simulink model "IEEE30_case"  (R2024b)
settings: Solver=FixedStepAuto  StartTime=0  StopTime=5  FixedStep=1e-7  RelTol=1e-3
values from neighbouring files (symbols this model uses):
  GFL_DFIG_7_C_bus = 0.08    [IEEE30_case_parameters.m]
  GFL_DFIG_7_D_mutual = 2.500000e+3    (= 2500)    [IEEE30_case_parameters.m]
  GFL_DFIG_7_f0 = 60    [IEEE30_case_parameters.m]
  GFL_DFIG_7_gPLLi = 3200    [IEEE30_case_parameters.m]
  GFL_DFIG_7_gPLLp = 650    [IEEE30_case_parameters.m]
  GFL_DFIG_7_H_WT = 0.4    [IEEE30_case_parameters.m]
  GFL_DFIG_7_Hg = 0.8    [IEEE30_case_parameters.m]
  GFL_DFIG_7_Igq_ref = 0    [IEEE30_case_parameters.m]
  GFL_DFIG_7_Ird_ref = 704.45696    [IEEE30_case_parameters.m]
  GFL_DFIG_7_KI_V = -300000    [IEEE30_case_parameters.m]
  GFL_DFIG_7_KP_V = -1000    [IEEE30_case_parameters.m]
  GFL_DFIG_7_Ksh = 1.254300e+4    (= 12543)    [IEEE30_case_parameters.m]
  GFL_DFIG_7_Lg = 0.000483    [IEEE30_case_parameters.m]
  GFL_DFIG_7_Lm_pu = 4    [IEEE30_case_parameters.m]
  GFL_DFIG_7_N = 100    [IEEE30_case_parameters.m]
  GFL_DFIG_7_p = 2    [IEEE30_case_parameters.m]
  GFL_DFIG_7_Pitch = 0    [IEEE30_case_parameters.m]
  GFL_DFIG_7_R = 44    [IEEE30_case_parameters.m]
  GFL_DFIG_7_Rg = 2.000000e-5    (= 2e-05)    [IEEE30_case_parameters.m]
  GFL_DFIG_7_rho = 1.225    [IEEE30_case_parameters.m]
  GFL_DFIG_7_rPLLi = 4500    [IEEE30_case_parameters.m]
  GFL_DFIG_7_rPLLp = 620    [IEEE30_case_parameters.m]
  GFL_DFIG_7_Rs_pu = 0.011    [IEEE30_case_parameters.m]
  GFL_DFIG_7_Sbase = 2.000000e+6    (= 2000000)    [IEEE30_case_parameters.m]
  GFL_DFIG_7_ugq_ref = 0    [IEEE30_case_parameters.m]
  GFL_DFIG_7_usd_ref = 0    [IEEE30_case_parameters.m]
  GFL_DFIG_7_Vbase = 690    [IEEE30_case_parameters.m]
  GFL_DFIG_7_Vdc_ref = 1200    [IEEE30_case_parameters.m]
  GFL_DFIG_7_wind = 12    [IEEE30_case_parameters.m]
  GFL_DFIG_7_wm_ref = 518.184209    [IEEE30_case_parameters.m]
  SG_D_13_D = 0.01056    [IEEE30_case_parameters.m]
  SG_D_13_EnableSaturation = 0    [IEEE30_case_parameters.m]
  SG_D_13_f0 = 60    [IEEE30_case_parameters.m]
  SG_D_13_H = 7.5    [IEEE30_case_parameters.m]
  SG_D_13_K_A = 20    [IEEE30_case_parameters.m]
  SG_D_13_K_E = 1.000000e+1    (= 10)    [IEEE30_case_parameters.m]
  SG_D_13_K_F = 2.363    [IEEE30_case_parameters.m]
  SG_D_13_K_s = 0.5    [IEEE30_case_parameters.m]
  SG_D_13_R_a = 0.001088    [IEEE30_case_parameters.m]
  SG_D_13_S_A = 1    [IEEE30_case_parameters.m]
  SG_D_13_S_B = 0.103    [IEEE30_case_parameters.m]
  SG_D_13_S_N = 10.659857    [IEEE30_case_parameters.m]
  SG_D_13_SpeedPara = 200    [IEEE30_case_parameters.m]
  SG_D_13_T_0 = 0.370163    [IEEE30_case_parameters.m]
  SG_D_13_T_1 = 0.3    [IEEE30_case_parameters.m]
  SG_D_13_T_2 = 0.05    [IEEE30_case_parameters.m]
  SG_D_13_T_3 = 0.02    [IEEE30_case_parameters.m]
  SG_D_13_T_4 = 0.005    [IEEE30_case_parameters.m]
  SG_D_13_T_A = 0.02    [IEEE30_case_parameters.m]
  SG_D_13_T_dd = 8.000000e+0    (= 8)    [IEEE30_case_parameters.m]
  SG_D_13_T_ddd = 0.04    [IEEE30_case_parameters.m]
  SG_D_13_T_E = 0.314    [IEEE30_case_parameters.m]
  SG_D_13_T_F = 0.35    [IEEE30_case_parameters.m]
  SG_D_13_T_qd = 0.8    [IEEE30_case_parameters.m]
  SG_D_13_T_qdd = 0.02    [IEEE30_case_parameters.m]
  SG_D_13_T_speed = 0.1    [IEEE30_case_parameters.m]
  SG_D_13_T_w = 0.5    [IEEE30_case_parameters.m]
  SG_D_13_V_ref = 1.696619    [IEEE30_case_parameters.m]
  SG_D_13_w_ref = 376.991118    [IEEE30_case_parameters.m]
  SG_D_13_x_d = 1.9    [IEEE30_case_parameters.m]
  SG_D_13_x_dd = 0.302    [IEEE30_case_parameters.m]
  SG_D_13_x_ddd = 0.204    [IEEE30_case_parameters.m]
  SG_D_13_x_l = 0.05    [IEEE30_case_parameters.m]
  SG_D_13_x_q = 1.3    [IEEE30_case_parameters.m]
  SG_D_13_x_qd = 0.5    [IEEE30_case_parameters.m]
  SG_D_13_x_qdd = 0.3    [IEEE30_case_parameters.m]
  SG_D_1_D = 0.01056    [IEEE30_case_parameters.m]
  SG_D_1_EnableSaturation = 0    [IEEE30_case_parameters.m]
  SG_D_1_f0 = 60    [IEEE30_case_parameters.m]
  SG_D_1_H = 7.5    [IEEE30_case_parameters.m]
  SG_D_1_K_A = 20    [IEEE30_case_parameters.m]
  SG_D_1_K_E = 1.000000e+1    (= 10)    [IEEE30_case_parameters.m]
  SG_D_1_K_F = 2.363    [IEEE30_case_parameters.m]
  SG_D_1_K_s = 0.5    [IEEE30_case_parameters.m]
  SG_D_1_R_a = 0.001088    [IEEE30_case_parameters.m]
  SG_D_1_S_A = 1    [IEEE30_case_parameters.m]
  SG_D_1_S_B = 0.103    [IEEE30_case_parameters.m]
  SG_D_1_S_N = 10.659857    [IEEE30_case_parameters.m]
  SG_D_1_SpeedPara = 200    [IEEE30_case_parameters.m]
  SG_D_1_T_0 = 0.259812    [IEEE30_case_parameters.m]
  SG_D_1_T_1 = 0.3    [IEEE30_case_parameters.m]
  SG_D_1_T_2 = 0.05    [IEEE30_case_parameters.m]
  SG_D_1_T_3 = 0.02    [IEEE30_case_parameters.m]
  SG_D_1_T_4 = 0.005    [IEEE30_case_parameters.m]
  SG_D_1_T_A = 0.02    [IEEE30_case_parameters.m]
  SG_D_1_T_dd = 8.000000e+0    (= 8)    [IEEE30_case_parameters.m]
  SG_D_1_T_ddd = 0.04    [IEEE30_case_parameters.m]
  SG_D_1_T_E = 0.314    [IEEE30_case_parameters.m]
  SG_D_1_T_F = 0.35    [IEEE30_case_parameters.m]
  SG_D_1_T_qd = 0.8    [IEEE30_case_parameters.m]
  SG_D_1_T_qdd = 0.02    [IEEE30_case_parameters.m]
  SG_D_1_T_speed = 0.1    [IEEE30_case_parameters.m]
  SG_D_1_T_w = 0.5    [IEEE30_case_parameters.m]
  SG_D_1_V_ref = 1.544107    [IEEE30_case_parameters.m]
  SG_D_1_w_ref = 376.991118    [IEEE30_case_parameters.m]
  SG_D_1_x_d = 1.9    [IEEE30_case_parameters.m]
  SG_D_1_x_dd = 0.302    [IEEE30_case_parameters.m]
  SG_D_1_x_ddd = 0.204    [IEEE30_case_parameters.m]
  SG_D_1_x_l = 0.05    [IEEE30_case_parameters.m]
  SG_D_1_x_q = 1.3    [IEEE30_case_parameters.m]
  SG_D_1_x_qd = 0.5    [IEEE30_case_parameters.m]
  SG_D_1_x_qdd = 0.3    [IEEE30_case_parameters.m]
  SG_D_22_D = 0.01056    [IEEE30_case_parameters.m]
  SG_D_22_EnableSaturation = 0    [IEEE30_case_parameters.m]
  SG_D_22_f0 = 60    [IEEE30_case_parameters.m]
  SG_D_22_H = 7.5    [IEEE30_case_parameters.m]
  SG_D_22_K_A = 20    [IEEE30_case_parameters.m]
  SG_D_22_K_E = 1.000000e+1    (= 10)    [IEEE30_case_parameters.m]
  SG_D_22_K_F = 2.363    [IEEE30_case_parameters.m]
  SG_D_22_K_s = 0.5    [IEEE30_case_parameters.m]
  SG_D_22_R_a = 0.001088    [IEEE30_case_parameters.m]
  SG_D_22_S_A = 1    [IEEE30_case_parameters.m]
  SG_D_22_S_B = 0.103    [IEEE30_case_parameters.m]
  SG_D_22_S_N = 10.659857    [IEEE30_case_parameters.m]
  SG_D_22_SpeedPara = 200    [IEEE30_case_parameters.m]
  SG_D_22_T_0 = 0.216121    [IEEE30_case_parameters.m]
  SG_D_22_T_1 = 0.3    [IEEE30_case_parameters.m]
  SG_D_22_T_2 = 0.05    [IEEE30_case_parameters.m]
  SG_D_22_T_3 = 0.02    [IEEE30_case_parameters.m]
  SG_D_22_T_4 = 0.005    [IEEE30_case_parameters.m]
  ... (+126 more)
(part 6 of 27)

== system IEEE30_case/AC_1/d_id_line_5_7_block ==
  note: d_id_line_5_7 in IEEE30_case
      | $376.991118430775\,\mathrm{iq}_{\mathrm{line},5,7}-157.07963267949\,\mathrm{id}_{\mathrm{line},5,7}+3141.59265358979\,\mathrm{vd}_{\mathrm{bus},5}-3141.59265358979\,\mathrm{vd}_{\mathrm{bus},7}$
      | Automatically generated on 2025-11-01 18:41:13 .
  State_id_line_5_7_f4de4 : Inport
  State_iq_line_5_7_abaf2 : Inport  Port=2
  State_vd_bus_5_fcd45 : Inport  Port=3
  State_vd_bus_7_ca274 : Inport  Port=4
  Add_3cebd : Sum
  Add_96d6b : Sum
  Constant_-157.07963267949_79139 : Constant  Value=-157.07963267949
  Constant_3141.59265358979_57f19 : Constant  Value=3141.59265358979
  Constant_3141.59265358979_dc5fb : Constant  Value=3141.59265358979
  Constant_376.991118430775_d7487 : Constant  Value=376.991118430775
  Product_17bef : Product
  Product_21c14 : Product
  Product_bd274 : Product
  Product_f508a : Product
  Subtract_98652 : Sum  Inputs=+-
  Blockout_d_id_line_5_7_7d91d : Outport
  wires:
  Subtract_98652/1 -> Blockout_d_id_line_5_7_7d91d/1
  State_id_line_5_7_f4de4/1 -> Product_17bef/2
  Constant_-157.07963267949_79139/1 -> Product_17bef/1
  Constant_376.991118430775_d7487/1 -> Product_bd274/1
  State_iq_line_5_7_abaf2/1 -> Product_bd274/2
  Product_bd274/1 -> Add_96d6b/2
  Product_17bef/1 -> Add_96d6b/1
  Product_f508a/1 -> Add_3cebd/2
  Constant_3141.59265358979_57f19/1 -> Product_f508a/1
  State_vd_bus_5_fcd45/1 -> Product_f508a/2
  Add_96d6b/1 -> Add_3cebd/1
  Product_21c14/1 -> Subtract_98652/2
  Constant_3141.59265358979_dc5fb/1 -> Product_21c14/1
  State_vd_bus_7_ca274/1 -> Product_21c14/2
  Add_3cebd/1 -> Subtract_98652/1

== system IEEE30_case/AC_1/d_id_line_6_10_block ==
  note: d_id_line_6_10 in IEEE30_case
      | $376.991118430775\,\mathrm{iq}_{\mathrm{line},6,10}+673.198425769241\,\mathrm{vd}_{\mathrm{bus},6}-673.198425769241\,\mathrm{vd}_{\mathrm{bus},10}$
      | Automatically generated on 2025-11-01 18:41:23 .
  State_iq_line_6_10_1e2b8 : Inport
  State_vd_bus_10_6889c : Inport  Port=2
  State_vd_bus_6_f8a31 : Inport  Port=3
  Add_cf162 : Sum
  Constant_376.991118430775_5db38 : Constant  Value=376.991118430775
  Constant_673.198425769241_4baa2 : Constant  Value=673.198425769241
  Constant_673.198425769241_5d573 : Constant  Value=673.198425769241
  Product_2d753 : Product
  Product_3532c : Product
  Product_b0b85 : Product
  Subtract_eeeb7 : Sum  Inputs=+-
  Blockout_d_id_line_6_10_40498 : Outport
  wires:
  Constant_376.991118430775_5db38/1 -> Product_2d753/1
  Constant_673.198425769241_5d573/1 -> Product_b0b85/1
  State_iq_line_6_10_1e2b8/1 -> Product_2d753/2
  Constant_673.198425769241_4baa2/1 -> Product_3532c/1
  Product_3532c/1 -> Subtract_eeeb7/2
  State_vd_bus_10_6889c/1 -> Product_3532c/2
  Product_2d753/1 -> Subtract_eeeb7/1
  State_vd_bus_6_f8a31/1 -> Product_b0b85/2
  Subtract_eeeb7/1 -> Add_cf162/1
  Product_b0b85/1 -> Add_cf162/2
  Add_cf162/1 -> Blockout_d_id_line_6_10_40498/1

== system IEEE30_case/AC_1/d_id_line_6_28_block ==
  note: d_id_line_6_28 in IEEE30_case
      | $376.991118430775\,\mathrm{iq}_{\mathrm{line},6,28}-125.663706143592\,\mathrm{id}_{\mathrm{line},6,28}+6283.18530717959\,\mathrm{vd}_{\mathrm{bus},6}-6283.18530717959\,\mathrm{vd}_{\mathrm{bus},28}$
      | Automatically generated on 2025-11-01 18:42:30 .
  State_id_line_6_28_16dd7 : Inport
  State_iq_line_6_28_4e6de : Inport  Port=2
  State_vd_bus_28_34661 : Inport  Port=3
  State_vd_bus_6_24f43 : Inport  Port=4
  Add_91382 : Sum
  Add_d7cc6 : Sum
  Constant_-125.663706143592_673b1 : Constant  Value=-125.663706143592
  Constant_376.991118430775_83a0d : Constant  Value=376.991118430775
  Constant_6283.18530717959_21113 : Constant  Value=6283.18530717959
  Constant_6283.18530717959_269c0 : Constant  Value=6283.18530717959
  Product_6c6ef : Product
  Product_d631f : Product
  Product_ea0c3 : Product
  Product_ec862 : Product
  Subtract_8b6c5 : Sum  Inputs=+-
  Blockout_d_id_line_6_28_3a173 : Outport
  wires:
  Constant_-125.663706143592_673b1/1 -> Product_d631f/1
  Constant_376.991118430775_83a0d/1 -> Product_ea0c3/1
  Product_ea0c3/1 -> Add_d7cc6/2
  State_id_line_6_28_16dd7/1 -> Product_d631f/2
  Add_91382/1 -> Blockout_d_id_line_6_28_3a173/1
  State_iq_line_6_28_4e6de/1 -> Product_ea0c3/2
  Product_d631f/1 -> Add_d7cc6/1
  Product_6c6ef/1 -> Subtract_8b6c5/2
  Constant_6283.18530717959_269c0/1 -> Product_6c6ef/1
  State_vd_bus_28_34661/1 -> Product_6c6ef/2
  Add_d7cc6/1 -> Subtract_8b6c5/1
  Product_ec862/1 -> Add_91382/2
  Constant_6283.18530717959_21113/1 -> Product_ec862/1
  State_vd_bus_6_24f43/1 -> Product_ec862/2
  Subtract_8b6c5/1 -> Add_91382/1

== system IEEE30_case/AC_1/d_id_line_6_7_block ==
  note: d_id_line_6_7 in IEEE30_case
      | $376.991118430775\,\mathrm{iq}_{\mathrm{line},6,7}-141.371669411541\,\mathrm{id}_{\mathrm{line},6,7}+4712.38898038469\,\mathrm{vd}_{\mathrm{bus},6}-4712.38898038469\,\mathrm{vd}_{\mathrm{bus},7}$
      | Automatically generated on 2025-11-01 18:41:16 .
  State_id_line_6_7_795b3 : Inport
  State_iq_line_6_7_8098b : Inport  Port=2
  State_vd_bus_6_7185e : Inport  Port=3
  State_vd_bus_7_fcdb6 : Inport  Port=4
  Add_20df1 : Sum
  Add_5e0cb : Sum
  Constant_-141.371669411541_b0a47 : Constant  Value=-141.371669411541
  Constant_376.991118430775_4adcf : Constant  Value=376.991118430775
  Constant_4712.38898038469_28790 : Constant  Value=4712.38898038469
  Constant_4712.38898038469_75038 : Constant  Value=4712.38898038469
  Product_b6763 : Product
  Product_dac56 : Product
  Product_e27ef : Product
  Product_fbe98 : Product
  Subtract_3d01d : Sum  Inputs=+-
  Blockout_d_id_line_6_7_5bfdb : Outport
  wires:
  Constant_-141.371669411541_b0a47/1 -> Product_fbe98/1
  State_id_line_6_7_795b3/1 -> Product_fbe98/2
  Constant_376.991118430775_4adcf/1 -> Product_b6763/1
  Product_b6763/1 -> Add_5e0cb/2
  State_iq_line_6_7_8098b/1 -> Product_b6763/2
  Product_fbe98/1 -> Add_5e0cb/1
  Constant_4712.38898038469_28790/1 -> Product_e27ef/1
  State_vd_bus_6_7185e/1 -> Product_e27ef/2
  Add_5e0cb/1 -> Add_20df1/1
  Product_e27ef/1 -> Add_20df1/2
  Product_dac56/1 -> Subtract_3d01d/2
  Constant_4712.38898038469_75038/1 -> Product_dac56/1
  State_vd_bus_7_fcdb6/1 -> Product_dac56/2
  Add_20df1/1 -> Subtract_3d01d/1
  Subtract_3d01d/1 -> Blockout_d_id_line_6_7_5bfdb/1

== system IEEE30_case/AC_1/d_id_line_6_8_block ==
  note: d_id_line_6_8 in IEEE30_case
      | $376.991118430775\,\mathrm{iq}_{\mathrm{line},6,8}-94.2477796076938\,\mathrm{id}_{\mathrm{line},6,8}+9424.77796076938\,\mathrm{vd}_{\mathrm{bus},6}-9424.77796076938\,\mathrm{vd}_{\mathrm{bus},8}$
      | Automatically generated on 2025-11-01 18:41:18 .
  State_id_line_6_8_be2c2 : Inport
  State_iq_line_6_8_15cb0 : Inport  Port=2
  State_vd_bus_6_a2a00 : Inport  Port=3
  State_vd_bus_8_3fe16 : Inport  Port=4
  Add_21824 : Sum
  Add_44597 : Sum
  Constant_-94.2477796076938_c506f : Constant  Value=-94.2477796076938
  Constant_376.991118430775_5cbac : Constant  Value=376.991118430775
  Constant_9424.77796076938_a2f7d : Constant  Value=9424.77796076938
  Constant_9424.77796076938_c3a88 : Constant  Value=9424.77796076938
  Product_448dc : Product
  Product_52dc7 : Product
  Product_5c49d : Product
  Product_d96d0 : Product
  Subtract_76e2a : Sum  Inputs=+-
  Blockout_d_id_line_6_8_230ec : Outport
  wires:
  State_vd_bus_6_a2a00/1 -> Product_448dc/2
  Constant_-94.2477796076938_c506f/1 -> Product_d96d0/1
  Product_448dc/1 -> Add_21824/2
  Constant_9424.77796076938_a2f7d/1 -> Product_448dc/1
  State_id_line_6_8_be2c2/1 -> Product_d96d0/2
  Constant_376.991118430775_5cbac/1 -> Product_52dc7/1
  Product_52dc7/1 -> Add_44597/2
  State_iq_line_6_8_15cb0/1 -> Product_52dc7/2
  Product_5c49d/1 -> Subtract_76e2a/2
  Constant_9424.77796076938_c3a88/1 -> Product_5c49d/1
  Product_d96d0/1 -> Add_44597/1
  Add_44597/1 -> Add_21824/1
  State_vd_bus_8_3fe16/1 -> Product_5c49d/2
  Add_21824/1 -> Subtract_76e2a/1
  Subtract_76e2a/1 -> Blockout_d_id_line_6_8_230ec/1

== system IEEE30_case/AC_1/d_id_line_6_9_block ==
  note: d_id_line_6_9 in IEEE30_case
      | $376.991118430775\,\mathrm{iq}_{\mathrm{line},6,9}+1795.19580205131\,\mathrm{vd}_{\mathrm{bus},6}-1795.19580205131\,\mathrm{vd}_{\mathrm{bus},9}$
      | Automatically generated on 2025-11-01 18:41:21 .
  State_iq_line_6_9_a3af3 : Inport
  State_vd_bus_6_dd441 : Inport  Port=2
  State_vd_bus_9_1e8eb : Inport  Port=3
  Add_a457a : Sum
  Constant_1795.19580205131_21e41 : Constant  Value=1795.19580205131
  Constant_1795.19580205131_4f3db : Constant  Value=1795.19580205131
  Constant_376.991118430775_846aa : Constant  Value=376.991118430775
  Product_8da75 : Product
  Product_af589 : Product
  Product_bd41a : Product
  Subtract_faf1e : Sum  Inputs=+-
  Blockout_d_id_line_6_9_67e91 : Outport
  wires:
  Constant_1795.19580205131_21e41/1 -> Product_8da75/1
  Product_bd41a/1 -> Add_a457a/1
  Constant_376.991118430775_846aa/1 -> Product_bd41a/1
  State_iq_line_6_9_a3af3/1 -> Product_bd41a/2
  Constant_1795.19580205131_4f3db/1 -> Product_af589/1
  Product_af589/1 -> Add_a457a/2
  State_vd_bus_6_dd441/1 -> Product_af589/2
  State_vd_bus_9_1e8eb/1 -> Product_8da75/2
  Add_a457a/1 -> Subtract_faf1e/1
  Product_8da75/1 -> Subtract_faf1e/2
  Subtract_faf1e/1 -> Blockout_d_id_line_6_9_67e91/1

== system IEEE30_case/AC_1/d_id_line_8_28_block ==
  note: d_id_line_8_28 in IEEE30_case
      | $376.991118430775\,\mathrm{iq}_{\mathrm{line},8,28}-113.097335529233\,\mathrm{id}_{\mathrm{line},8,28}+1884.95559215388\,\mathrm{vd}_{\mathrm{bus},8}-1884.95559215388\,\mathrm{vd}_{\mathrm{bus},28}$
      | Automatically generated on 2025-11-01 18:42:27 .
  State_id_line_8_28_e35e6 : Inport
  State_iq_line_8_28_05745 : Inport  Port=2
  State_vd_bus_28_83ac0 : Inport  Port=3
  State_vd_bus_8_26ad6 : Inport  Port=4
  Add_4ec08 : Sum
  Add_5c3f1 : Sum
  Constant_-113.097335529233_90aea : Constant  Value=-113.097335529233
  Constant_1884.95559215388_94dcd : Constant  Value=1884.95559215388
  Constant_1884.95559215388_9cb5d : Constant  Value=1884.95559215388
  Constant_376.991118430775_979c0 : Constant  Value=376.991118430775
  Product_3587f : Product
  Product_8fb7e : Product
  Product_9a9ee : Product
  Product_e88f7 : Product
  Subtract_b3740 : Sum  Inputs=+-
  Blockout_d_id_line_8_28_c2b8a : Outport
  wires:
  Constant_-113.097335529233_90aea/1 -> Product_9a9ee/1
  Constant_1884.95559215388_94dcd/1 -> Product_e88f7/1
  Add_5c3f1/1 -> Blockout_d_id_line_8_28_c2b8a/1
  State_id_line_8_28_e35e6/1 -> Product_9a9ee/2
  Constant_376.991118430775_979c0/1 -> Product_8fb7e/1
  Product_8fb7e/1 -> Add_4ec08/2
  State_iq_line_8_28_05745/1 -> Product_8fb7e/2
  Product_9a9ee/1 -> Add_4ec08/1
  State_vd_bus_28_83ac0/1 -> Product_e88f7/2
  Add_4ec08/1 -> Subtract_b3740/1
  Product_e88f7/1 -> Subtract_b3740/2
  Product_3587f/1 -> Add_5c3f1/2
  Constant_1884.95559215388_9cb5d/1 -> Product_3587f/1
  State_vd_bus_8_26ad6/1 -> Product_3587f/2
  Subtract_b3740/1 -> Add_5c3f1/1

== system IEEE30_case/AC_1/d_id_line_9_10_block ==
  note: d_id_line_9_10 in IEEE30_case
      | $376.991118430775\,\mathrm{iq}_{\mathrm{line},9,10}+3427.19198573432\,\mathrm{vd}_{\mathrm{bus},9}-3427.19198573432\,\mathrm{vd}_{\mathrm{bus},10}$
      | Automatically generated on 2025-11-01 18:41:27 .
  State_iq_line_9_10_60482 : Inport
  State_vd_bus_10_163ea : Inport  Port=2
  State_vd_bus_9_a12d0 : Inport  Port=3
  Add_dcdd8 : Sum
  Constant_3427.19198573432_49acf : Constant  Value=3427.19198573432
  Constant_3427.19198573432_8d0a7 : Constant  Value=3427.19198573432
  Constant_376.991118430775_2c152 : Constant  Value=376.991118430775
  Product_9eddb : Product
  Product_b6cde : Product
  Product_eef34 : Product
  Subtract_03e25 : Sum  Inputs=+-
  Blockout_d_id_line_9_10_c8100 : Outport
  wires:
  State_iq_line_9_10_60482/1 -> Product_9eddb/2
  Constant_376.991118430775_2c152/1 -> Product_9eddb/1
  Constant_3427.19198573432_8d0a7/1 -> Product_eef34/1
  Product_eef34/1 -> Subtract_03e25/2
  State_vd_bus_10_163ea/1 -> Product_eef34/2
  Product_9eddb/1 -> Subtract_03e25/1
  Constant_3427.19198573432_49acf/1 -> Product_b6cde/1
  State_vd_bus_9_a12d0/1 -> Product_b6cde/2
  Subtract_03e25/1 -> Add_dcdd8/1
  Product_b6cde/1 -> Add_dcdd8/2
  Add_dcdd8/1 -> Blockout_d_id_line_9_10_c8100/1

== system IEEE30_case/AC_1/d_id_line_9_11_block ==
  note: d_id_line_9_11 in IEEE30_case
      | $376.991118430775\,\mathrm{iq}_{\mathrm{line},9,11}+1795.19580205131\,\mathrm{vd}_{\mathrm{bus},9}-1795.19580205131\,\mathrm{vd}_{\mathrm{bus},11}$
      | Automatically generated on 2025-11-01 18:41:25 .
  State_iq_line_9_11_d1a32 : Inport
  State_vd_bus_11_30158 : Inport  Port=2
  State_vd_bus_9_653b8 : Inport  Port=3
  Add_d11a9 : Sum
  Constant_1795.19580205131_64bcc : Constant  Value=1795.19580205131
  Constant_1795.19580205131_d59c3 : Constant  Value=1795.19580205131
  Constant_376.991118430775_3b578 : Constant  Value=376.991118430775
  Product_1e074 : Product
  Product_1fdd9 : Product
  Product_4efb2 : Product
  Subtract_8d526 : Sum  Inputs=+-
  Blockout_d_id_line_9_11_6700a : Outport
  wires:
  Constant_376.991118430775_3b578/1 -> Product_4efb2/1
  Constant_1795.19580205131_d59c3/1 -> Product_1fdd9/1
  Product_1fdd9/1 -> Subtract_8d526/2
  State_iq_line_9_11_d1a32/1 -> Product_4efb2/2
  State_vd_bus_11_30158/1 -> Product_1fdd9/2
  Product_4efb2/1 -> Subtract_8d526/1
  Constant_1795.19580205131_64bcc/1 -> Product_1e074/1
  State_vd_bus_9_653b8/1 -> Product_1e074/2
  Subtract_8d526/1 -> Add_d11a9/1
  Product_1e074/1 -> Add_d11a9/2
  Add_d11a9/1 -> Blockout_d_id_line_9_11_6700a/1

== system IEEE30_case/AC_1/d_id_load_10_block ==
  note: d_id_load_10 in IEEE30_case
      | $376.991118430775\,\mathrm{iq}_{\mathrm{load},10}-1093.27424344925\,\mathrm{id}_{\mathrm{load},10}+73.2156181903037\,\mathrm{vd}_{\mathrm{bus},10}$
      | Automatically generated on 2025-11-01 18:40:25 .
  State_id_load_10_b4421 : Inport
  State_iq_load_10_46bbe : Inport  Port=2
  State_vd_bus_10_876fd : Inport  Port=3
  Add_683f6 : Sum
  Add_8289f : Sum
  Constant_-1093.27424344925_8b95d : Constant  Value=-1093.27424344925
  Constant_376.991118430775_85e18 : Constant  Value=376.991118430775
  Constant_73.2156181903037_3ac9c : Constant  Value=73.2156181903037
  Product_21a59 : Product
  Product_23bbe : Product
  Product_24f80 : Product
  Blockout_d_id_load_10_a9a8b : Outport
  wires:
  Constant_-1093.27424344925_8b95d/1 -> Product_24f80/1
  Constant_376.991118430775_85e18/1 -> Product_21a59/1
  Product_21a59/1 -> Add_8289f/2
  Product_24f80/1 -> Add_8289f/1
  State_id_load_10_b4421/1 -> Product_24f80/2
  State_iq_load_10_46bbe/1 -> Product_21a59/2
  Product_23bbe/1 -> Add_683f6/2
  Constant_73.2156181903037_3ac9c/1 -> Product_23bbe/1
  State_vd_bus_10_876fd/1 -> Product_23bbe/2
  Add_8289f/1 -> Add_683f6/1
  Add_683f6/1 -> Blockout_d_id_load_10_a9a8b/1

== system IEEE30_case/AC_1/d_id_load_12_block ==
  note: d_id_load_12 in IEEE30_case
      | $376.991118430775\,\mathrm{iq}_{\mathrm{load},12}-562.973403523291\,\mathrm{id}_{\mathrm{load},12}+94.0406333232708\,\mathrm{vd}_{\mathrm{bus},12}$
      | Automatically generated on 2025-11-01 18:40:27 .
  State_id_load_12_7246e : Inport
  State_iq_load_12_5d0f3 : Inport  Port=2
  State_vd_bus_12_e073f : Inport  Port=3
  Add_15efc : Sum
  Add_f0d24 : Sum
  Constant_-562.973403523291_16ce0 : Constant  Value=-562.973403523291
  Constant_376.991118430775_26874 : Constant  Value=376.991118430775
  Constant_94.0406333232708_30ced : Constant  Value=94.0406333232708
  Product_2d4c6 : Product
  Product_385f8 : Product
  Product_9dcd7 : Product
  Blockout_d_id_load_12_82ad0 : Outport
  wires:
  Constant_-562.973403523291_16ce0/1 -> Product_385f8/1
  Product_385f8/1 -> Add_15efc/1
  State_id_load_12_7246e/1 -> Product_385f8/2
  Constant_376.991118430775_26874/1 -> Product_9dcd7/1
  Product_9dcd7/1 -> Add_15efc/2
  State_iq_load_12_5d0f3/1 -> Product_9dcd7/2
  Product_2d4c6/1 -> Add_f0d24/2
  Constant_94.0406333232708_30ced/1 -> Product_2d4c6/1
  State_vd_bus_12_e073f/1 -> Product_2d4c6/2
  Add_15efc/1 -> Add_f0d24/1
  Add_f0d24/1 -> Blockout_d_id_load_12_82ad0/1

== system IEEE30_case/AC_1/d_id_load_14_block ==
  note: d_id_load_14 in IEEE30_case
      | $376.991118430775\,\mathrm{iq}_{\mathrm{load},14}-1460.84058391925\,\mathrm{id}_{\mathrm{load},14}+101.272894526084\,\mathrm{vd}_{\mathrm{bus},14}$
      | Automatically generated on 2025-11-01 18:40:30 .
  State_id_load_14_cc3a3 : Inport
  State_iq_load_14_d649f : Inport  Port=2
  State_vd_bus_14_f08fd : Inport  Port=3
  Add_0838c : Sum
  Add_4ad40 : Sum
  Constant_-1460.84058391925_2a859 : Constant  Value=-1460.84058391925
  Constant_101.272894526084_890bb : Constant  Value=101.272894526084
  Constant_376.991118430775_aab37 : Constant  Value=376.991118430775
  Product_31438 : Product
  Product_944f5 : Product
  Product_a5863 : Product
  Blockout_d_id_load_14_6d751 : Outport
  wires:
  Constant_-1460.84058391925_2a859/1 -> Product_31438/1
  Product_31438/1 -> Add_4ad40/1
  State_id_load_14_cc3a3/1 -> Product_31438/2
  Constant_376.991118430775_aab37/1 -> Product_944f5/1
  Product_944f5/1 -> Add_4ad40/2
  Product_a5863/1 -> Add_0838c/2
  Constant_101.272894526084_890bb/1 -> Product_a5863/1
  State_iq_load_14_d649f/1 -> Product_944f5/2
  Add_0838c/1 -> Blockout_d_id_load_14_6d751/1
  State_vd_bus_14_f08fd/1 -> Product_a5863/2
  Add_4ad40/1 -> Add_0838c/1

== system IEEE30_case/AC_1/d_id_load_15_block ==
  note: d_id_load_15 in IEEE30_case
      | $376.991118430775\,\mathrm{iq}_{\mathrm{load},15}-1236.53086845294\,\mathrm{id}_{\mathrm{load},15}+115.335827789783\,\mathrm{vd}_{\mathrm{bus},15}$
      | Automatically generated on 2025-11-01 18:40:32 .
  State_id_load_15_eb719 : Inport
  State_iq_load_15_a3946 : Inport  Port=2
  State_vd_bus_15_8a842 : Inport  Port=3
  Add_5f190 : Sum
  Add_ffceb : Sum
  Constant_-1236.53086845294_1de0b : Constant  Value=-1236.53086845294
  Constant_115.335827789783_e0e0e : Constant  Value=115.335827789783
  Constant_376.991118430775_a00d5 : Constant  Value=376.991118430775
  Product_d7855 : Product
  Product_d9c37 : Product
  Product_f5b16 : Product
  Blockout_d_id_load_15_10a9e : Outport
  wires:
  State_vd_bus_15_8a842/1 -> Product_f5b16/2
  Add_ffceb/1 -> Add_5f190/1
  Constant_-1236.53086845294_1de0b/1 -> Product_d7855/1
  Product_f5b16/1 -> Add_5f190/2
  Constant_115.335827789783_e0e0e/1 -> Product_f5b16/1
  Product_d7855/1 -> Add_ffceb/1
  State_id_load_15_eb719/1 -> Product_d7855/2
  Constant_376.991118430775_a00d5/1 -> Product_d9c37/1
  Product_d9c37/1 -> Add_ffceb/2
  State_iq_load_15_a3946/1 -> Product_d9c37/2
  Add_5f190/1 -> Blockout_d_id_load_15_10a9e/1

== system IEEE30_case/AC_1/d_id_load_16_block ==
  note: d_id_load_16 in IEEE30_case
      | $376.991118430775\,\mathrm{iq}_{\mathrm{load},16}-733.038285837618\,\mathrm{id}_{\mathrm{load},16}+33.9601202098734\,\mathrm{vd}_{\mathrm{bus},16}$
      | Automatically generated on 2025-11-01 18:40:34 .
  State_id_load_16_b19cd : Inport
  State_iq_load_16_b414b : Inport  Port=2
  State_vd_bus_16_dbff6 : Inport  Port=3
  Add_04344 : Sum
  Add_c11be : Sum
  Constant_-733.038285837618_5814f : Constant  Value=-733.038285837618
  Constant_33.9601202098734_4dcff : Constant  Value=33.9601202098734
  Constant_376.991118430775_a0c4a : Constant  Value=376.991118430775
  Product_052c1 : Product
  Product_a73ff : Product
  Product_e285b : Product
  Blockout_d_id_load_16_4c50d : Outport
  wires:
  Constant_-733.038285837618_5814f/1 -> Product_a73ff/1
  Constant_376.991118430775_a0c4a/1 -> Product_052c1/1
  Product_052c1/1 -> Add_c11be/2
  Product_a73ff/1 -> Add_c11be/1
  State_id_load_16_b19cd/1 -> Product_a73ff/2
  State_iq_load_16_b414b/1 -> Product_052c1/2
  Product_e285b/1 -> Add_04344/2
  Constant_33.9601202098734_4dcff/1 -> Product_e285b/1
  Add_04344/1 -> Blockout_d_id_load_16_4c50d/1
  State_vd_bus_16_dbff6/1 -> Product_e285b/2
  Add_c11be/1 -> Add_04344/1

== system IEEE30_case/AC_1/d_id_load_17_block ==
  note: d_id_load_17 in IEEE30_case
      | $376.991118430775\,\mathrm{iq}_{\mathrm{load},17}-584.986218254651\,\mathrm{id}_{\mathrm{load},17}+78.0853999068988\,\mathrm{vd}_{\mathrm{bus},17}$
      | Automatically generated on 2025-11-01 18:40:36 .
  State_id_load_17_a4ece : Inport
  State_iq_load_17_ca59a : Inport  Port=2
  State_vd_bus_17_34bc4 : Inport  Port=3
  Add_b66f2 : Sum
  Add_f0f0b : Sum
  Constant_-584.986218254651_7f0eb : Constant  Value=-584.986218254651
  Constant_376.991118430775_c7146 : Constant  Value=376.991118430775
  Constant_78.0853999068988_505df : Constant  Value=78.0853999068988
  Product_113aa : Product
  Product_75b41 : Product
  Product_d00df : Product
  Blockout_d_id_load_17_000e5 : Outport
  wires:
  Constant_-584.986218254651_7f0eb/1 -> Product_75b41/1
  Product_75b41/1 -> Add_b66f2/1
  State_id_load_17_a4ece/1 -> Product_75b41/2
  Constant_376.991118430775_c7146/1 -> Product_d00df/1
  Product_d00df/1 -> Add_b66f2/2
  State_iq_load_17_ca59a/1 -> Product_d00df/2
  Product_113aa/1 -> Add_f0f0b/2
  Constant_78.0853999068988_505df/1 -> Product_113aa/1
  State_vd_bus_17_34bc4/1 -> Product_113aa/2
  Add_b66f2/1 -> Add_f0f0b/1
  Add_f0f0b/1 -> Blockout_d_id_load_17_000e5/1

== system IEEE30_case/AC_1/d_id_load_18_block ==
  note: d_id_load_18 in IEEE30_case
      | $376.991118430775\,\mathrm{iq}_{\mathrm{load},18}-1340.41286553164\,\mathrm{id}_{\mathrm{load},18}+49.3520450041255\,\mathrm{vd}_{\mathrm{bus},18}$
      | Automatically generated on 2025-11-01 18:40:38 .
  State_id_load_18_c255f : Inport
  State_iq_load_18_e520e : Inport  Port=2
  State_vd_bus_18_bf8f3 : Inport  Port=3
  Add_045e5 : Sum
  Add_5e28f : Sum
  Constant_-1340.41286553164_81c67 : Constant  Value=-1340.41286553164
  Constant_376.991118430775_9c70f : Constant  Value=376.991118430775
  Constant_49.3520450041255_59f5b : Constant  Value=49.3520450041255
  Product_50b44 : Product
  Product_a97c5 : Product
  Product_c1ec3 : Product
  Blockout_d_id_load_18_3083b : Outport
  wires:
  Constant_-1340.41286553164_81c67/1 -> Product_a97c5/1
  Product_a97c5/1 -> Add_5e28f/1
  State_id_load_18_c255f/1 -> Product_a97c5/2
  Constant_376.991118430775_9c70f/1 -> Product_c1ec3/1
  Product_c1ec3/1 -> Add_5e28f/2
  Product_50b44/1 -> Add_045e5/2
  Constant_49.3520450041255_59f5b/1 -> Product_50b44/1
  State_iq_load_18_e520e/1 -> Product_c1ec3/2
  State_vd_bus_18_bf8f3/1 -> Product_50b44/2
  Add_5e28f/1 -> Add_045e5/1
  Add_045e5/1 -> Blockout_d_id_load_18_3083b/1

== system IEEE30_case/AC_1/d_id_load_19_block ==
  note: d_id_load_19 in IEEE30_case
      | $376.991118430775\,\mathrm{iq}_{\mathrm{load},19}-1053.35753679187\,\mathrm{id}_{\mathrm{load},19}+121.151749063551\,\mathrm{vd}_{\mathrm{bus},19}$
      | Automatically generated on 2025-11-01 18:40:40 .
  State_id_load_19_86caa : Inport
  State_iq_load_19_76cc3 : Inport  Port=2
  State_vd_bus_19_07a12 : Inport  Port=3
  Add_39f41 : Sum
  Add_8d624 : Sum
  Constant_-1053.35753679187_bafe0 : Constant  Value=-1053.35753679187
  Constant_121.151749063551_084ae : Constant  Value=121.151749063551
  Constant_376.991118430775_456e5 : Constant  Value=376.991118430775
  Product_003ce : Product
  Product_1d94f : Product
  Product_8f6a5 : Product
  Blockout_d_id_load_19_c7816 : Outport
  wires:
  State_vd_bus_19_07a12/1 -> Product_8f6a5/2
  Constant_-1053.35753679187_bafe0/1 -> Product_1d94f/1
  Product_8f6a5/1 -> Add_8d624/2
  Constant_121.151749063551_084ae/1 -> Product_8f6a5/1
  Product_1d94f/1 -> Add_39f41/1
  State_id_load_19_86caa/1 -> Product_1d94f/2
  Constant_376.991118430775_456e5/1 -> Product_003ce/1
  Product_003ce/1 -> Add_39f41/2
  State_iq_load_19_76cc3/1 -> Product_003ce/2
  Add_39f41/1 -> Add_8d624/1
  Add_8d624/1 -> Blockout_d_id_load_19_c7816/1

== system IEEE30_case/AC_1/d_id_load_20_block ==
  note: d_id_load_20 in IEEE30_case
      | $376.991118430775\,\mathrm{iq}_{\mathrm{load},20}-1184.82922935387\,\mathrm{id}_{\mathrm{load},20}+30.5607236833912\,\mathrm{vd}_{\mathrm{bus},20}$
      | Automatically generated on 2025-11-01 18:40:42 .
  State_id_load_20_93d05 : Inport
  State_iq_load_20_02020 : Inport  Port=2
  State_vd_bus_20_a40d3 : Inport  Port=3
  Add_3d016 : Sum
  Add_73b62 : Sum
  Constant_-1184.82922935387_94f65 : Constant  Value=-1184.82922935387
  Constant_30.5607236833912_571fa : Constant  Value=30.5607236833912
  Constant_376.991118430775_c13cd : Constant  Value=376.991118430775
  Product_3ef52 : Product
  Product_51416 : Product
  Product_7406c : Product
  Blockout_d_id_load_20_0f852 : Outport
  wires:
  Constant_-1184.82922935387_94f65/1 -> Product_51416/1
  Constant_376.991118430775_c13cd/1 -> Product_3ef52/1
  Product_3ef52/1 -> Add_73b62/2
  Product_51416/1 -> Add_73b62/1
  State_id_load_20_93d05/1 -> Product_51416/2
  State_iq_load_20_02020/1 -> Product_3ef52/2
  Product_7406c/1 -> Add_3d016/2
  Constant_30.5607236833912_571fa/1 -> Product_7406c/1
  Add_3d016/1 -> Blockout_d_id_load_20_0f852/1
  State_vd_bus_20_a40d3/1 -> Product_7406c/2
  Add_73b62/1 -> Add_3d016/1

== system IEEE30_case/AC_1/d_id_load_21_block ==
  note: d_id_load_21 in IEEE30_case
      | $376.991118430775\,\mathrm{iq}_{\mathrm{load},21}-589.048622548086\,\mathrm{id}_{\mathrm{load},21}+147.248668081812\,\mathrm{vd}_{\mathrm{bus},21}$
      | Automatically generated on 2025-11-01 18:40:44 .
  State_id_load_21_69a18 : Inport
  State_iq_load_21_49e98 : Inport  Port=2
  State_vd_bus_21_5dea6 : Inport  Port=3
  Add_80ae7 : Sum
  Add_a054e : Sum
  Constant_-589.048622548086_4f999 : Constant  Value=-589.048622548086
  Constant_147.248668081812_4d1f4 : Constant  Value=147.248668081812
  Constant_376.991118430775_edf1b : Constant  Value=376.991118430775
  Product_106cf : Product
  Product_1caf2 : Product
  Product_768ed : Product
  Blockout_d_id_load_21_f09db : Outport
  wires:
  Constant_-589.048622548086_4f999/1 -> Product_768ed/1
  Product_768ed/1 -> Add_80ae7/1
  State_id_load_21_69a18/1 -> Product_768ed/2
  Constant_376.991118430775_edf1b/1 -> Product_106cf/1
  Product_106cf/1 -> Add_80ae7/2
  State_iq_load_21_49e98/1 -> Product_106cf/2
  Product_1caf2/1 -> Add_a054e/2
  Constant_147.248668081812_4d1f4/1 -> Product_1caf2/1
  State_vd_bus_21_5dea6/1 -> Product_1caf2/2
  Add_80ae7/1 -> Add_a054e/1
  Add_a054e/1 -> Blockout_d_id_load_21_f09db/1

== system IEEE30_case/AC_1/d_id_load_23_block ==
  note: d_id_load_23 in IEEE30_case
      | $376.991118430775\,\mathrm{iq}_{\mathrm{load},23}-753.98223686155\,\mathrm{id}_{\mathrm{load},23}+30.159289474462\,\mathrm{vd}_{\mathrm{bus},23}$
      | Automatically generated on 2025-11-01 18:40:46 .
  State_id_load_23_139dd : Inport
  State_iq_load_23_9ed9d : Inport  Port=2
  State_vd_bus_23_3d25c : Inport  Port=3
  Add_cb4a1 : Sum
  Add_fda1a : Sum
  Constant_-753.98223686155_779b8 : Constant  Value=-753.98223686155
  Constant_30.159289474462_e23cc : Constant  Value=30.159289474462
  Constant_376.991118430775_7c271 : Constant  Value=376.991118430775
  Product_85ff3 : Product
  Product_e9dc7 : Product
  Product_f749f : Product
  Blockout_d_id_load_23_0d04d : Outport
  wires:
  Constant_-753.98223686155_779b8/1 -> Product_85ff3/1
  Product_85ff3/1 -> Add_cb4a1/1
  State_id_load_23_139dd/1 -> Product_85ff3/2
  Constant_376.991118430775_7c271/1 -> Product_e9dc7/1
  Product_e9dc7/1 -> Add_cb4a1/2
  Product_f749f/1 -> Add_fda1a/2
  Constant_30.159289474462_e23cc/1 -> Product_f749f/1
  State_iq_load_23_9ed9d/1 -> Product_e9dc7/2
  State_vd_bus_23_3d25c/1 -> Product_f749f/2
  Add_fda1a/1 -> Blockout_d_id_load_23_0d04d/1
  Add_cb4a1/1 -> Add_fda1a/1

== system IEEE30_case/AC_1/d_id_load_24_block ==
  note: d_id_load_24 in IEEE30_case
      | $376.991118430775\,\mathrm{iq}_{\mathrm{load},24}-489.525780648917\,\mathrm{id}_{\mathrm{load},24}+69.4256561190419\,\mathrm{vd}_{\mathrm{bus},24}$
      | Automatically generated on 2025-11-01 18:40:48 .
  State_id_load_24_1ae10 : Inport
  State_iq_load_24_33ce7 : Inport  Port=2
  State_vd_bus_24_e8709 : Inport  Port=3
  Add_2b358 : Sum
  Add_f3861 : Sum
  Constant_-489.525780648917_3d885 : Constant  Value=-489.525780648917
  Constant_376.991118430775_5f561 : Constant  Value=376.991118430775
  Constant_69.4256561190419_6c15a : Constant  Value=69.4256561190419
  Product_11a3b : Product
  Product_24c41 : Product
  Product_5935c : Product
  Blockout_d_id_load_24_7bbe2 : Outport
  wires:
  State_vd_bus_24_e8709/1 -> Product_11a3b/2
  Constant_-489.525780648917_3d885/1 -> Product_24c41/1
  Product_11a3b/1 -> Add_2b358/2
  Constant_69.4256561190419_6c15a/1 -> Product_11a3b/1
  Product_24c41/1 -> Add_f3861/1
  State_id_load_24_1ae10/1 -> Product_24c41/2
  Constant_376.991118430775_5f561/1 -> Product_5935c/1
  Product_5935c/1 -> Add_f3861/2
  State_iq_load_24_33ce7/1 -> Product_5935c/2
  Add_f3861/1 -> Add_2b358/1
  Add_2b358/1 -> Blockout_d_id_load_24_7bbe2/1

== system IEEE30_case/AC_1/d_id_load_26_block ==
  note: d_id_load_26 in IEEE30_case
      | $376.991118430775\,\mathrm{iq}_{\mathrm{load},26}-573.682136742484\,\mathrm{id}_{\mathrm{load},26}+30.4177344988829\,\mathrm{vd}_{\mathrm{bus},26}$
      | Automatically generated on 2025-11-01 18:40:50 .
  State_id_load_26_7d329 : Inport
  State_iq_load_26_8de5f : Inport  Port=2
  State_vd_bus_26_1ef7d : Inport  Port=3
  Add_a8ac2 : Sum
  Add_ab0a7 : Sum
  Constant_-573.682136742484_70732 : Constant  Value=-573.682136742484
  Constant_30.4177344988829_4842c : Constant  Value=30.4177344988829
  Constant_376.991118430775_fb0b4 : Constant  Value=376.991118430775
  Product_3e15b : Product
  Product_4fa69 : Product
  Product_c716b : Product
  Blockout_d_id_load_26_29eef : Outport
  wires:
  Constant_-573.682136742484_70732/1 -> Product_4fa69/1
  Constant_376.991118430775_fb0b4/1 -> Product_c716b/1
  Product_c716b/1 -> Add_a8ac2/2
  Product_4fa69/1 -> Add_a8ac2/1
  State_id_load_26_7d329/1 -> Product_4fa69/2
  State_iq_load_26_8de5f/1 -> Product_c716b/2
  Product_3e15b/1 -> Add_ab0a7/2
  Constant_30.4177344988829_4842c/1 -> Product_3e15b/1
  State_vd_bus_26_1ef7d/1 -> Product_3e15b/2
  Add_a8ac2/1 -> Add_ab0a7/1
  Add_ab0a7/1 -> Blockout_d_id_load_26_29eef/1

== system IEEE30_case/AC_1/d_id_load_29_block ==
  note: d_id_load_29 in IEEE30_case
      | $376.991118430775\,\mathrm{iq}_{\mathrm{load},29}-1005.30964914873\,\mathrm{id}_{\mathrm{load},29}+28.6786928048477\,\mathrm{vd}_{\mathrm{bus},29}$
      | Automatically generated on 2025-11-01 18:40:52 .
  State_id_load_29_75998 : Inport
  State_iq_load_29_726f9 : Inport  Port=2
  State_vd_bus_29_01a46 : Inport  Port=3
  Add_096fd : Sum
  Add_c4333 : Sum
  Constant_-1005.30964914873_4c6ee : Constant  Value=-1005.30964914873
  Constant_28.6786928048477_c193b : Constant  Value=28.6786928048477
  Constant_376.991118430775_3c60a : Constant  Value=376.991118430775
  Product_6b013 : Product
  Product_791a8 : Product
  Product_c42d3 : Product
  Blockout_d_id_load_29_ee930 : Outport
  wires:
  Add_096fd/1 -> Add_c4333/1
  Constant_-1005.30964914873_4c6ee/1 -> Product_c42d3/1
  Product_c42d3/1 -> Add_096fd/1
  State_id_load_29_75998/1 -> Product_c42d3/2
  Constant_376.991118430775_3c60a/1 -> Product_791a8/1
  Product_791a8/1 -> Add_096fd/2
  State_iq_load_29_726f9/1 -> Product_791a8/2
  Product_6b013/1 -> Add_c4333/2
  Constant_28.6786928048477_c193b/1 -> Product_6b013/1
  State_vd_bus_29_01a46/1 -> Product_6b013/2
  Add_c4333/1 -> Blockout_d_id_load_29_ee930/1

== system IEEE30_case/AC_1/d_id_load_2_block ==
  note: d_id_load_2 in IEEE30_case
      | $376.991118430775\,\mathrm{iq}_{\mathrm{load},2}-644.150178736049\,\mathrm{id}_{\mathrm{load},2}+187.658460826431\,\mathrm{vd}_{\mathrm{bus},2}$
      | Automatically generated on 2025-11-01 18:40:14 .
  State_id_load_2_b9eb3 : Inport
  State_iq_load_2_16be9 : Inport  Port=2
  State_vd_bus_2_46ad8 : Inport  Port=3
  Add_0a498 : Sum
  Add_c8c31 : Sum
  Constant_-644.150178736049_6a6d4 : Constant  Value=-644.150178736049
  Constant_187.658460826431_55d7c : Constant  Value=187.658460826431
  Constant_376.991118430775_2d4f7 : Constant  Value=376.991118430775
  Product_03ad6 : Product
  Product_a3185 : Product
  Product_f3371 : Product
  Blockout_d_id_load_2_a0af3 : Outport
  wires:
  State_vd_bus_2_46ad8/1 -> Product_a3185/2
  Constant_-644.150178736049_6a6d4/1 -> Product_03ad6/1
  Product_03ad6/1 -> Add_0a498/1
  Product_a3185/1 -> Add_c8c31/2
  Constant_187.658460826431_55d7c/1 -> Product_a3185/1
  State_id_load_2_b9eb3/1 -> Product_03ad6/2
  Constant_376.991118430775_2d4f7/1 -> Product_f3371/1
  Product_f3371/1 -> Add_0a498/2
  State_iq_load_2_16be9/1 -> Product_f3371/2
  Add_0a498/1 -> Add_c8c31/1
  Add_c8c31/1 -> Blockout_d_id_load_2_a0af3/1

== system IEEE30_case/AC_1/d_id_load_30_block ==
  note: d_id_load_30 in IEEE30_case
      | $376.991118430775\,\mathrm{iq}_{\mathrm{load},30}-2103.21360808748\,\mathrm{id}_{\mathrm{load},30}+245.627822821845\,\mathrm{vd}_{\mathrm{bus},30}$
      | Automatically generated on 2025-11-01 18:40:54 .
  State_id_load_30_f5eec : Inport
  State_iq_load_30_241a5 : Inport  Port=2
  State_vd_bus_30_c111a : Inport  Port=3
  Add_b54c5 : Sum
  Add_f898c : Sum
  Constant_-2103.21360808748_a3447 : Constant  Value=-2103.21360808748
  Constant_245.627822821845_0e239 : Constant  Value=245.627822821845
  Constant_376.991118430775_fc958 : Constant  Value=376.991118430775
  Product_5ed96 : Product
  Product_700f9 : Product
  Product_a45fa : Product
  Blockout_d_id_load_30_6a7a7 : Outport
  wires:
  Constant_-2103.21360808748_a3447/1 -> Product_a45fa/1
  Constant_376.991118430775_fc958/1 -> Product_5ed96/1
  Product_5ed96/1 -> Add_b54c5/2
  Product_a45fa/1 -> Add_b54c5/1
  State_id_load_30_f5eec/1 -> Product_a45fa/2
  State_iq_load_30_241a5/1 -> Product_5ed96/2
  Product_700f9/1 -> Add_f898c/2
  Constant_245.627822821845_0e239/1 -> Product_700f9/1
  Add_f898c/1 -> Blockout_d_id_load_30_6a7a7/1
  State_vd_bus_30_c111a/1 -> Product_700f9/2
  Add_b54c5/1 -> Add_f898c/1

== system IEEE30_case/AC_1/d_id_load_3_block ==
  note: d_id_load_3 in IEEE30_case
      | $376.991118430775\,\mathrm{iq}_{\mathrm{load},3}-753.98223686155\,\mathrm{id}_{\mathrm{load},3}+23.4020092990225\,\mathrm{vd}_{\mathrm{bus},3}$
      | Automatically generated on 2025-11-01 18:40:17 .
  State_id_load_3_6ca3f : Inport
  State_iq_load_3_e3dcb : Inport  Port=2
  State_vd_bus_3_703c2 : Inport  Port=3
  Add_a2206 : Sum
  Add_e9327 : Sum
  Constant_-753.98223686155_27bf7 : Constant  Value=-753.98223686155
  Constant_23.4020092990225_cfb13 : Constant  Value=23.4020092990225
  Constant_376.991118430775_2770c : Constant  Value=376.991118430775
  Product_30cb6 : Product
  Product_5007e : Product
  Product_59e16 : Product
  Blockout_d_id_load_3_d01d9 : Outport
  wires:
  Constant_-753.98223686155_27bf7/1 -> Product_5007e/1
  Constant_376.991118430775_2770c/1 -> Product_30cb6/1
  Product_30cb6/1 -> Add_a2206/2
  Product_5007e/1 -> Add_a2206/1
  State_id_load_3_6ca3f/1 -> Product_5007e/2
  State_iq_load_3_e3dcb/1 -> Product_30cb6/2
  Product_59e16/1 -> Add_e9327/2
  Constant_23.4020092990225_cfb13/1 -> Product_59e16/1
  State_vd_bus_3_703c2/1 -> Product_59e16/2
  Add_a2206/1 -> Add_e9327/1
  Add_e9327/1 -> Blockout_d_id_load_3_d01d9/1

== system IEEE30_case/AC_1/d_id_load_4_block ==
  note: d_id_load_4 in IEEE30_case
      | $376.991118430775\,\mathrm{iq}_{\mathrm{load},4}-1790.70781254618\,\mathrm{id}_{\mathrm{load},4}+147.957809890804\,\mathrm{vd}_{\mathrm{bus},4}$
      | Automatically generated on 2025-11-01 18:40:19 .
  State_id_load_4_a067e : Inport
  State_iq_load_4_59598 : Inport  Port=2
  State_vd_bus_4_a96c2 : Inport  Port=3
  Add_28b14 : Sum
  Add_2e701 : Sum
  Constant_-1790.70781254618_4a751 : Constant  Value=-1790.70781254618
  Constant_147.957809890804_b436d : Constant  Value=147.957809890804
  Constant_376.991118430775_a92b6 : Constant  Value=376.991118430775
  Product_6b4e9 : Product
  Product_ee5ea : Product
  Product_f31c8 : Product
  Blockout_d_id_load_4_41d2b : Outport
  wires:
  Add_28b14/1 -> Add_2e701/1
  Constant_-1790.70781254618_4a751/1 -> Product_f31c8/1
  Product_f31c8/1 -> Add_28b14/1
  State_id_load_4_a067e/1 -> Product_f31c8/2
  Constant_376.991118430775_a92b6/1 -> Product_ee5ea/1
  Product_ee5ea/1 -> Add_28b14/2
  State_iq_load_4_59598/1 -> Product_ee5ea/2
  Product_6b4e9/1 -> Add_2e701/2
  Constant_147.957809890804_b436d/1 -> Product_6b4e9/1
  State_vd_bus_4_a96c2/1 -> Product_6b4e9/2
  Add_2e701/1 -> Blockout_d_id_load_4_41d2b/1

== system IEEE30_case/AC_1/d_id_load_7_block ==
  note: d_id_load_7 in IEEE30_case
      | $376.991118430775\,\mathrm{iq}_{\mathrm{load},7}-1134.43198940637\,\mathrm{id}_{\mathrm{load},7}+441.543140918512\,\mathrm{vd}_{\mathrm{bus},7}$
      | Automatically generated on 2025-11-01 18:40:21 .
  State_id_load_7_59ac3 : Inport
  State_iq_load_7_25d21 : Inport  Port=2
  State_vd_bus_7_efc9a : Inport  Port=3
  Add_04136 : Sum
  Add_741b9 : Sum
  Constant_-1134.43198940637_835a7 : Constant  Value=-1134.43198940637
  Constant_376.991118430775_d91d4 : Constant  Value=376.991118430775
  Constant_441.543140918512_82739 : Constant  Value=441.543140918512
  Product_275c3 : Product
  Product_2927f : Product
  Product_c6f97 : Product
  Blockout_d_id_load_7_06d7e : Outport
  wires:
  Constant_-1134.43198940637_835a7/1 -> Product_c6f97/1
  Product_c6f97/1 -> Add_04136/1
  State_id_load_7_59ac3/1 -> Product_c6f97/2
  Constant_376.991118430775_d91d4/1 -> Product_2927f/1
  Product_2927f/1 -> Add_04136/2
  Product_275c3/1 -> Add_741b9/2
  Constant_441.543140918512_82739/1 -> Product_275c3/1
  State_iq_load_7_25d21/1 -> Product_2927f/2
  Add_741b9/1 -> Blockout_d_id_load_7_06d7e/1
  State_vd_bus_7_efc9a/1 -> Product_275c3/2
  Add_04136/1 -> Add_741b9/1

== system IEEE30_case/AC_1/d_id_load_8_block ==
  note: d_id_load_8 in IEEE30_case
      | $376.991118430775\,\mathrm{iq}_{\mathrm{load},8}-376.991118430775\,\mathrm{id}_{\mathrm{load},8}+245.118316875829\,\mathrm{vd}_{\mathrm{bus},8}$
      | Automatically generated on 2025-11-01 18:40:23 .
  State_id_load_8_d111e : Inport
  State_iq_load_8_8935f : Inport  Port=2
  State_vd_bus_8_e6dd7 : Inport  Port=3
  Add_157b4 : Sum
  Add_7efb3 : Sum
  Constant_-376.991118430775_0c58f : Constant  Value=-376.991118430775
  Constant_245.118316875829_f0525 : Constant  Value=245.118316875829
  Constant_376.991118430775_eff81 : Constant  Value=376.991118430775
  Product_53c12 : Product
  Product_9e446 : Product
  Product_d8fa2 : Product
  Blockout_d_id_load_8_0e169 : Outport
  wires:
  State_vd_bus_8_e6dd7/1 -> Product_53c12/2
  Constant_-376.991118430775_0c58f/1 -> Product_9e446/1
  Product_53c12/1 -> Add_157b4/2
  Constant_245.118316875829_f0525/1 -> Product_53c12/1
  Product_9e446/1 -> Add_7efb3/1
  State_id_load_8_d111e/1 -> Product_9e446/2
  Constant_376.991118430775_eff81/1 -> Product_d8fa2/1
  Product_d8fa2/1 -> Add_7efb3/2
  State_iq_load_8_8935f/1 -> Product_d8fa2/2
  Add_7efb3/1 -> Add_157b4/1
  Add_157b4/1 -> Blockout_d_id_load_8_0e169/1

== system IEEE30_case/AC_1/d_iq_line_10_17_block ==
  note: d_iq_line_10_17 in IEEE30_case
      | $4712.38898038469\,\mathrm{vq}_{\mathrm{bus},10}-141.371669411541\,\mathrm{iq}_{\mathrm{line},10,17}-376.991118430775\,\mathrm{id}_{\mathrm{line},10,17}-4712.38898038469\,\mathrm{vq}_{\mathrm{bus},17}$
      | Automatically generated on 2025-11-01 18:41:55 .
  State_id_line_10_17_8e75b : Inport
  State_iq_line_10_17_a9ea7 : Inport  Port=2
  State_vq_bus_10_bd672 : Inport  Port=3
  State_vq_bus_17_4f180 : Inport  Port=4
  Add_0cd68 : Sum
  Constant_-376.991118430775_acb6c : Constant  Value=-376.991118430775
  Constant_141.371669411541_599f2 : Constant  Value=141.371669411541
  Constant_4712.38898038469_08db1 : Constant  Value=4712.38898038469
  Constant_4712.38898038469_b6468 : Constant  Value=4712.38898038469
  Product_1cbe7 : Product
  Product_28120 : Product
  Product_ebec5 : Product
  Product_ef122 : Product
  Subtract_6d114 : Sum  Inputs=+-
  Subtract_d64b7 : Sum  Inputs=+-
  Blockout_d_iq_line_10_17_34a6b : Outport
  wires:
  Constant_-376.991118430775_acb6c/1 -> Product_1cbe7/1
  Product_1cbe7/1 -> Subtract_6d114/1
  State_id_line_10_17_8e75b/1 -> Product_1cbe7/2
  Constant_141.371669411541_599f2/1 -> Product_28120/1
  Product_28120/1 -> Subtract_6d114/2
  Product_ef122/1 -> Add_0cd68/2
  Constant_4712.38898038469_08db1/1 -> Product_ef122/1
  State_iq_line_10_17_a9ea7/1 -> Product_28120/2
  State_vq_bus_10_bd672/1 -> Product_ef122/2
  Subtract_6d114/1 -> Add_0cd68/1
  Constant_4712.38898038469_b6468/1 -> Product_ebec5/1
  Add_0cd68/1 -> Subtract_d64b7/1
  State_vq_bus_17_4f180/1 -> Product_ebec5/2
  Product_ebec5/1 -> Subtract_d64b7/2
  Subtract_d64b7/1 -> Blockout_d_iq_line_10_17_34a6b/1

== system IEEE30_case/AC_1/d_iq_line_10_20_block ==
  note: d_iq_line_10_20 in IEEE30_case
      | $1795.19580205131\,\mathrm{vq}_{\mathrm{bus},10}-161.567622184618\,\mathrm{iq}_{\mathrm{line},10,20}-376.991118430775\,\mathrm{id}_{\mathrm{line},10,20}-1795.19580205131\,\mathrm{vq}_{\mathrm{bus},20}$
      | Automatically generated on 2025-11-01 18:41:53 .
  State_id_line_10_20_31cef : Inport
  State_iq_line_10_20_af332 : Inport  Port=2
  State_vq_bus_10_01ccf : Inport  Port=3
  State_vq_bus_20_32cb1 : Inport  Port=4
  Add_e9c2c : Sum
  Constant_-376.991118430775_4839d : Constant  Value=-376.991118430775
  Constant_161.567622184618_c0e5d : Constant  Value=161.567622184618
  Constant_1795.19580205131_335c2 : Constant  Value=1795.19580205131
  Constant_1795.19580205131_4b625 : Constant  Value=1795.19580205131
  Product_3ca2d : Product
  Product_a7271 : Product
  Product_c1a61 : Product
  Product_d1909 : Product
  Subtract_6cf01 : Sum  Inputs=+-
  Subtract_cb49c : Sum  Inputs=+-
  Blockout_d_iq_line_10_20_deb13 : Outport
  wires:
  Product_a7271/1 -> Subtract_6cf01/1
  Constant_-376.991118430775_4839d/1 -> Product_a7271/1
  State_id_line_10_20_31cef/1 -> Product_a7271/2
  Constant_161.567622184618_c0e5d/1 -> Product_c1a61/1
  Product_c1a61/1 -> Subtract_6cf01/2
  State_iq_line_10_20_af332/1 -> Product_c1a61/2
  Subtract_6cf01/1 -> Add_e9c2c/1
  Constant_1795.19580205131_4b625/1 -> Product_3ca2d/1
  State_vq_bus_10_01ccf/1 -> Product_3ca2d/2
  Product_3ca2d/1 -> Add_e9c2c/2
  Product_d1909/1 -> Subtract_cb49c/2
  Constant_1795.19580205131_335c2/1 -> Product_d1909/1
  State_vq_bus_20_32cb1/1 -> Product_d1909/2
  Add_e9c2c/1 -> Subtract_cb49c/1
  Subtract_cb49c/1 -> Blockout_d_iq_line_10_20_deb13/1
